simulink model "PEM_Electrolyzer_Complete"  (R2023b)
settings: Solver=VariableStepAuto  StartTime=0.0  StopTime=100  RelTol=1e-3
settings Model: Creator=Admin  LastModifiedBy=Admin
settings DataIOCC: SaveFormat=StructureWithTime

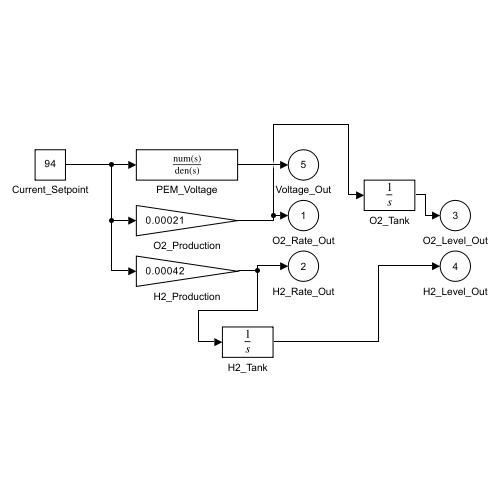
[thumbnail: Simulink's stored preview of the top-level diagram]
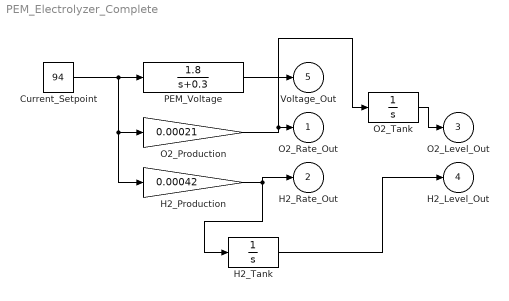
== system PEM_Electrolyzer_Complete ==
  Current_Setpoint : Constant  Value=94
  H2_Production : Gain  Gain=0.00042
  H2_Tank : Integrator  InitialCondition=10
  O2_Production : Gain  Gain=0.00021
  O2_Tank : Integrator  InitialCondition=10
  PEM_Voltage : TransferFcn  Numerator=[1.8]  Denominator=[1 0.3]
  O2_Rate_Out : Outport
  H2_Rate_Out : Outport  Port=2
  O2_Level_Out : Outport  Port=3
  H2_Level_Out : Outport  Port=4
  Voltage_Out : Outport  Port=5
  wires:
  Current_Setpoint/1 -> H2_Production/1, O2_Production/1, PEM_Voltage/1
  PEM_Voltage/1 -> Voltage_Out/1
  O2_Production/1 -> O2_Rate_Out/1, O2_Tank/1
  H2_Production/1 -> H2_Rate_Out/1, H2_Tank/1
  O2_Tank/1 -> O2_Level_Out/1
  H2_Tank/1 -> H2_Level_Out/1
